simulink model "Simulator_BlockDiagram"  (R2020a)
settings: Solver=FixedStepAuto  StartTime=0.0  StopTime=20  FixedStep=dt  RelTol=1e-3
values from neighbouring files (symbols this model uses):
  Beq = 60    [SimulationParam.m]    (also in SimulationParameters.m; abc_ws.mat; kalmanSS.m; kalmanSSHumInput.m)
  damping_d = 0.001    [SimulationParam.m]    (also in SimulationParameters.m; abc_ws.mat = 0.770835010154; kalmanSSHumInput.m = 0.9)
  dt = 0.001    [SimulationParam.m]    (also in SimulationParameters.m; kalmanSS.m; kalmanSSHumInput.m)
  epos_Ki = 1.190    (= 1.19)    [SimulationParam.m]    (also in SimulationParameters.m; abc_ws.mat; kalmanSSHumInput.m)
  epos_Kp = 11.900    (= 11.9)    [SimulationParam.m]    (also in SimulationParameters.m; abc_ws.mat; kalmanSSHumInput.m)
  Ja = 0.47    [SimulationParam.m]    (also in SimulationParameters.m; abc_ws.mat; kalmanSS.m; kalmanSSHumInput.m)
  Je = W*Le^2    (= 0.88498313856)    [SimulationParam.m]    (also in SimulationParameters.m; abc_ws.mat; kalmanSS.m; kalmanSSHumInput.m)
  Jh = 0.0437    [SimulationParam.m]    (also in SimulationParameters.m; abc_ws.mat; kalmanSS.m; kalmanSSHumInput.m)
  k_bar = 1 - stiffness_d/Ks    (= 0.993269230769)    [SimulationParam.m]    (also in SimulationParameters.m)
  Ka = Ks/20    (= 5.2)    [SimulationParam.m]    (also in SimulationParameters.m; abc_ws.mat = 1387.6; kalmanSS.m = 1387.6; kalmanSSHumInput.m = 800)
  Ks = 104    [SimulationParam.m]    (also in SimulationParameters.m; abc_ws.mat; kalmanSS.m; kalmanSSHumInput.m)
  Le = 0.432    [SimulationParam.m]    (also in SimulationParameters.m; abc_ws.mat; kalmanSS.m; kalmanSSHumInput.m)
  stiffness_d = 0.7    [SimulationParam.m]    (also in SimulationParameters.m; abc_ws.mat = 14.0803237251; kalmanSSHumInput.m = 3.874)
  We = W*g    (= 46.5037717323)    [SimulationParam.m]    (also in SimulationParameters.m; abc_ws.mat; kalmanSS.m; kalmanSSHumInput.m)
libraries: simulink x4, simulink_extras x2, dspstat3 x1
settings Model: Creator=leona  LastModifiedBy=leona
settings DataIOCC: SaveFormat=StructureWithTime  SaveOutput=off  SignalLogging=off  DSMLogging=off  SaveTime=off  ReturnWorkspaceOutputs=off

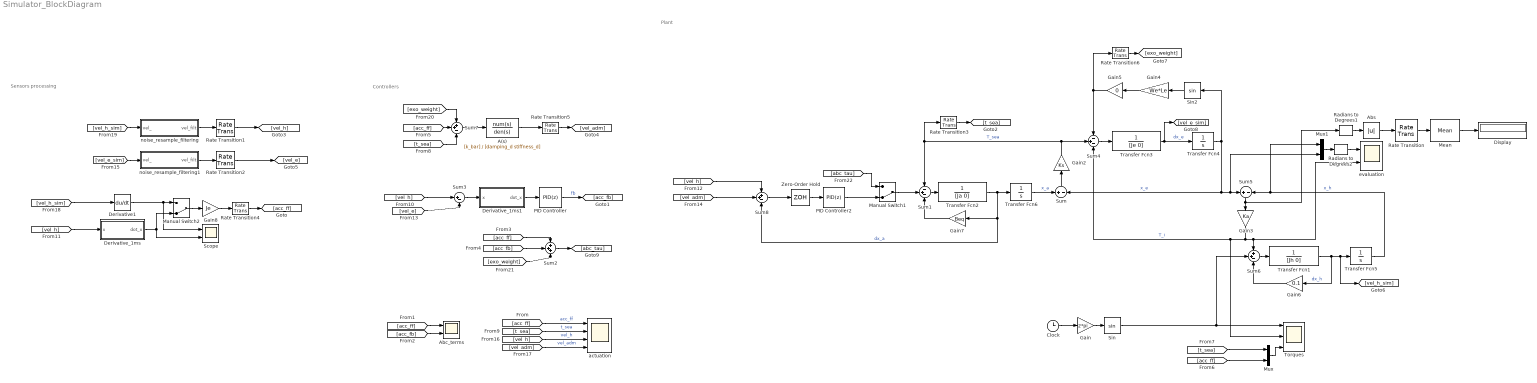
== system Simulator_BlockDiagram ==
  note: Plant
  note: Controllers
  note: Sensors processing
  A(s) : TransferFcn  Numerator=[k_bar]  Denominator=[damping_d stiffness_d]
  Abc_terms : Scope  NumInputPorts=2
  Abs : Abs
  Clock : Clock
  Derivative1 : Derivative
  Derivative_1ms : Subsystem
  Derivative_1ms1 : Subsystem
  Display : Display
  Gain : Gain  Gain=2*pi
  Gain2 : Gain  Gain=Ks
  Gain3 : Gain  Gain=Ka
  Gain4 : Gain  Gain=We*Le
  Gain5 : Gain  Gain=0
  Gain6 : Gain  Gain=0.1
  Gain7 : Gain  Gain=Beq
  Gain8 : Gain  Gain=Je
  Manual Switch1 : ManualSwitch  CurrentSetting=0
  Manual Switch2 : ManualSwitch  CurrentSetting=0
  Mean : dspstat3/Mean  run=on  InputProcessing=Columns as channels (frame based)  reset_popup=None  directionMode=Each column  dimension=1  roiEnable=off  roiType=Rectangles  roiPortion=Entire ROI  roiOutput=Individual statistics for each ROI  roiFlag=off  roundingMode=Floor  overflowMode=off  outputDataTypeStr=Inherit: Same as accumulator  outputMin=[]  outputMax=[]  outputLastDataTypeStr=Inherit: Same as accumulator
  Mux : Mux  Inputs=2
  Mux1 : Mux  Inputs=2
  PID Controller : simulink/Continuous/PID Controller  Controller=PID  Form=Parallel  TimeDomain=Discrete-time  UseExternalTs=off  SampleTime=dt  IntegratorMethod=Forward Euler  FilterMethod=Forward Euler  ControllerParametersSource=internal  P=.1  I=0  D=.01  UseFilter=off  N=100  TunerSelectOption=Transfer Function Based (PID Tuner App)  InitialConditionSource=internal  InitialConditionForIntegrator=0  InitialConditionForFilter=0  DifferentiatorICPrevScaledInput=0  ExternalReset=none  TrackingMode=off  Kt=1  LimitOutput=off  UpperSaturationLimit=inf  LowerSaturationLimit=-inf  LinearizeAsGain=on  AntiWindupMode=none  Kb=1  POutMin=[]  POutMax=[]  IOutMin=[]  IOutMax=[]  DOutMin=[]  DOutMax=[]  NOutMin=[]  NOutMax=[]  SumOutMin=[]  SumOutMax=[]  SaturationOutMin=[]  SaturationOutMax=[]  PParamMin=[]  PParamMax=[]  IParamMin=[]  IParamMax=[]  DParamMin=[]  DParamMax=[]  NParamMin=[]  NParamMax=[]  KbParamMin=[]  KbParamMax=[]  KtParamMin=[]  KtParamMax=[]  KbOutMin=[]  KbOutMax=[]  KtOutMin=[]  KtOutMax=[]  IntegratorOutMin=[]  IntegratorOutMax=[]  FilterOutMin=[]  FilterOutMax=[]  SumI1OutMin=[]  SumI1OutMax=[]  SumI2OutMin=[]  SumI2OutMax=[]  SumI3OutMin=[]  SumI3OutMax=[]  SumI4OutMin=[]  SumI4OutMax=[]  SumDOutMin=[]  SumDOutMax=[]  DifferentiatorOutMin=[]  DifferentiatorOutMax=[]  FilterDiffOutCoefMin=[]  FilterDiffOutCoefMax=[]  ReciprocalOutMin=[]  ReciprocalOutMax=[]  SumDenOutMin=[]  SumDenOutMax=[]  SumNumOutMin=[]  SumNumOutMax=[]  DivideOutMin=[]  DivideOutMax=[]  UdiffTsProdOutMin=[]  UdiffTsProdOutMax=[]  NTsProdOutMin=[]  NTsProdOutMax=[]  UintegralTsProdOutMin=[]  UintegralTsProdOutMax=[]  UngainTsProdOutMin=[]  UngainTsProdOutMax=[]  IntegratorContinuousStateAttributes=''  IntegratorStateMustResolveToSignalObject=off  IntegratorRTWStateStorageClass=Auto  FilterContinuousStateAttributes=''  FilterStateMustResolveToSignalObject=off  FilterRTWStateStorageClass=Auto  ParallelPVariant=InternalParameters  IdealPVariant=Disabled  IVariant=InternalParameters  DVariant=InternalParameters  IntegratorVariant=Discrete  SatVariant=Disabled  AWVariant=Passthrough  PCopyVariant=Disabled  TRVariant=Disabled  FdbkBlocksVariant=Forward  IdealPFdbkVariant=Disabled  SatFdbkVariant=Disabled  DerivativeFilterVariant=Differentiator  NVariant=Passthrough  NCopyVariant=Disabled_SignalSpec  FilterICVariant=InternalICsDifferentiator  IntegratorICVariant=InternalICs  ExternalResetVariant=Disabled  TRSumVariant=Passthrough  SumFdbkVariant=Disabled  SumVariant=Sum_PID  TsampFilterVariant=InternalTs  TsampNgainVariant=Passthrough  TsampIntegralVariant=Passthrough
  PID Controller2 : simulink/Continuous/PID Controller  Controller=PID  Form=Parallel  TimeDomain=Discrete-time  UseExternalTs=off  SampleTime=dt  IntegratorMethod=Forward Euler  FilterMethod=Forward Euler  ControllerParametersSource=internal  P=epos_Kp  I=epos_Ki  D=0  UseFilter=on  N=100  TunerSelectOption=Transfer Function Based (PID Tuner App)  InitialConditionSource=internal  InitialConditionForIntegrator=0  InitialConditionForFilter=0  DifferentiatorICPrevScaledInput=0  ExternalReset=none  TrackingMode=off  Kt=1  LimitOutput=off  UpperSaturationLimit=inf  LowerSaturationLimit=-inf  LinearizeAsGain=on  AntiWindupMode=none  Kb=1  POutMin=[]  POutMax=[]  IOutMin=[]  IOutMax=[]  DOutMin=[]  DOutMax=[]  NOutMin=[]  NOutMax=[]  SumOutMin=[]  SumOutMax=[]  SaturationOutMin=[]  SaturationOutMax=[]  PParamMin=[]  PParamMax=[]  IParamMin=[]  IParamMax=[]  DParamMin=[]  DParamMax=[]  NParamMin=[]  NParamMax=[]  KbParamMin=[]  KbParamMax=[]  KtParamMin=[]  KtParamMax=[]  KbOutMin=[]  KbOutMax=[]  KtOutMin=[]  KtOutMax=[]  IntegratorOutMin=[]  IntegratorOutMax=[]  FilterOutMin=[]  FilterOutMax=[]  SumI1OutMin=[]  SumI1OutMax=[]  SumI2OutMin=[]  SumI2OutMax=[]  SumI3OutMin=[]  SumI3OutMax=[]  SumI4OutMin=[]  SumI4OutMax=[]  SumDOutMin=[]  SumDOutMax=[]  DifferentiatorOutMin=[]  DifferentiatorOutMax=[]  FilterDiffOutCoefMin=[]  FilterDiffOutCoefMax=[]  ReciprocalOutMin=[]  ReciprocalOutMax=[]  SumDenOutMin=[]  SumDenOutMax=[]  SumNumOutMin=[]  SumNumOutMax=[]  DivideOutMin=[]  DivideOutMax=[]  UdiffTsProdOutMin=[]  UdiffTsProdOutMax=[]  NTsProdOutMin=[]  NTsProdOutMax=[]  UintegralTsProdOutMin=[]  UintegralTsProdOutMax=[]  UngainTsProdOutMin=[]  UngainTsProdOutMax=[]  IntegratorContinuousStateAttributes=''  IntegratorStateMustResolveToSignalObject=off  IntegratorRTWStateStorageClass=Auto  FilterContinuousStateAttributes=''  FilterStateMustResolveToSignalObject=off  FilterRTWStateStorageClass=Auto  ParallelPVariant=InternalParameters  IdealPVariant=Disabled  IVariant=InternalParameters  DVariant=InternalParameters  IntegratorVariant=Discrete  SatVariant=Disabled  AWVariant=Passthrough  PCopyVariant=Disabled  TRVariant=Disabled  FdbkBlocksVariant=Forward  IdealPFdbkVariant=Disabled  SatFdbkVariant=Disabled  DerivativeFilterVariant=ForwardEulerFilter  NVariant=InternalParameters  NCopyVariant=Disabled  FilterICVariant=InternalICsFilter  IntegratorICVariant=InternalICs  ExternalResetVariant=Disabled  TRSumVariant=Passthrough  SumFdbkVariant=Disabled  SumVariant=Sum_PID  TsampFilterVariant=InternalTs  TsampNgainVariant=Passthrough  TsampIntegralVariant=Passthrough
  Radians to Degrees1 : simulink_extras/Transformations/Radians to Degrees
  Radians to Degrees2 : simulink_extras/Transformations/Radians to Degrees
  Rate Transition{,1..6} (7 alike) : RateTransition  OutPortSampleTime=dt
  Scope : Scope  NumInputPorts=2
  Sin : Trigonometry
  Sin2 : Trigonometry
  Sum : Sum  Inputs=+-
  Sum1 : Sum  Inputs=-+-
  Sum2 : Sum  Inputs=+++
  Sum3 : Sum  Inputs=|+-
  Sum4 : Sum  Inputs=-+-
  Sum5 : Sum  Inputs=+-
  Sum6 : Sum  Inputs=++-
  Sum7 : Sum  Inputs=++-
  Sum8 : Sum  Inputs=++-
  Torques : Scope  NumInputPorts=3
  Transfer Fcn1 : TransferFcn  Denominator=[Jh 0]
  Transfer Fcn2 : TransferFcn  Denominator=[Ja 0]
  Transfer Fcn3 : TransferFcn  Denominator=[Je 0]
  Transfer Fcn4 : TransferFcn  Denominator=[1 0]
  Transfer Fcn5 : TransferFcn  Denominator=[1 0]
  Transfer Fcn6 : TransferFcn  Denominator=[1 0]
  Zero-Order Hold : ZeroOrderHold  SampleTime=-1
  actuation : Scope  NumInputPorts=4
  evaluation : Scope  NumInputPorts=2
  noise_resample_filtering : Subsystem
  noise_resample_filtering1 : Subsystem
  wires:
  Transfer Fcn6/1 -> Sum/1  "x_a"
  Derivative1/1 -> Scope/1, Manual Switch2/1
  Sum1/1 -> Transfer Fcn2/1
  Sum/1 -> Gain2/1
  Gain2/1 -> Sum4/2, Rate Transition3/1, Sum1/1  "T_sea"
  Sum3/1 -> Derivative_1ms1/1(x)
  Sum4/1 -> Transfer Fcn3/1
  Transfer Fcn4/1 -> Sin2/1, Mux1/2, Sum5/1, Sum/2  "x_e"
  Sin/1 -> Sum6/2, Torques/1
  Sum6/1 -> Transfer Fcn1/1
  Transfer Fcn5/1 -> Mux1/1, Sum5/2  "x_h"
  Sum5/1 -> Radians to Degrees1/1, Gain3/1
  Gain3/1 -> Sum4/3, Torques/2, Sum6/1, evaluation/2  "T_i"
  Transfer Fcn1/1 -> Gain6/1, [vel_h_sim], Transfer Fcn5/1  "dx_h"
  Manual Switch2/1 -> Gain8/1
  Transfer Fcn2/1 -> Sum8/3, Gain7/1, Transfer Fcn6/1  "dx_a"
  Clock/1 -> Gain/1
  Gain/1 -> Sin/1
  Derivative_1ms1/1(dot_x) -> PID Controller/1
  Mux/1 -> Torques/3
  Sum7/1 -> A(s)/1
  Sum8/1 -> Zero-Order Hold/1
  Gain4/1 -> Gain5/1
  Gain5/1 -> Sum4/1, Rate Transition6/1
  Sin2/1 -> Gain4/1
  A(s)/1 -> Rate Transition5/1
  Gain7/1 -> Sum1/3
  Gain6/1 -> Sum6/3
  Radians to Degrees2/1 -> evaluation/1
  Mux1/1 -> Radians to Degrees2/1
  Radians to Degrees1/1 -> Abs/1
  Abs/1 -> Rate Transition/1
  Rate Transition/1 -> Mean/1
  Mean/1 -> Display/1
  [acc_ff] -> Abc_terms/1
  PID Controller/1 -> [acc_fb]  "fb"
  [acc_fb] -> Abc_terms/2
  [acc_ff] -> Sum2/1
  [acc_fb] -> Sum2/2
  [acc_ff] -> Sum7/2
  [acc_ff] -> Mux/2
  [t_sea] -> Sum7/3
  [t_sea] -> Mux/1
  [acc_ff] -> actuation/1  "acc_ff"
  [t_sea] -> actuation/2  "t_sea"
  [vel_h] -> Sum3/1
  [vel_e] -> Sum3/2
  [vel_adm] -> Sum8/2
  [vel_adm] -> actuation/4  "vel_adm"
  [vel_h] -> actuation/3  "vel_h"
  Transfer Fcn3/1 -> [vel_e_sim], Transfer Fcn4/1  "dx_e"
  Gain8/1 -> Rate Transition4/1
  Derivative_1ms/1(dot_x) -> Scope/2, Manual Switch2/2
  [vel_h] -> Sum8/1
  [vel_h] -> Derivative_1ms/1(x)
  noise_resample_filtering/1(vel_filt) -> Rate Transition1/1
  Rate Transition1/1 -> [vel_h]
  noise_resample_filtering1/1(vel_filt) -> Rate Transition2/1
  Rate Transition2/1 -> [vel_e]
  [vel_h_sim] -> Derivative1/1
  [vel_e_sim] -> noise_resample_filtering1/1(vel_)
  [vel_h_sim] -> noise_resample_filtering/1(vel_)
  Rate Transition3/1 -> [t_sea]
  Rate Transition4/1 -> [acc_ff]
  Rate Transition5/1 -> [vel_adm]
  [exo_weight] -> Sum7/1
  Rate Transition6/1 -> [exo_weight]
  Zero-Order Hold/1 -> PID Controller2/1
  Manual Switch1/1 -> Sum1/2
  PID Controller2/1 -> Manual Switch1/2
  [exo_weight] -> Sum2/3
  Sum2/1 -> [abc_tau]
  [abc_tau] -> Manual Switch1/1

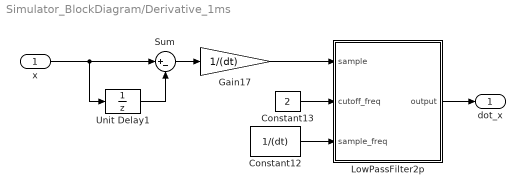
== system Simulator_BlockDiagram/Derivative_1ms ==
  x : Inport
  Constant12 : Constant  Value=1/(dt)
  Constant13 : Constant  Value=2
  Gain17 : Gain  Gain=1/(dt)
  LowPassFilter2p : Subsystem
  Sum : Sum  Inputs=|+-
  Unit Delay1 : UnitDelay  SampleTime=-1  HasFrameUpgradeWarning=on
  dot_x : Outport
  wires:
  Unit Delay1/1 -> Sum/2
  Sum/1 -> Gain17/1
  Gain17/1 -> LowPassFilter2p/1(sample)
  LowPassFilter2p/1(output) -> dot_x/1
  Constant12/1 -> LowPassFilter2p/3(sample_freq)
  x/1 -> Unit Delay1/1, Sum/1
  Constant13/1 -> LowPassFilter2p/2(cutoff_freq)

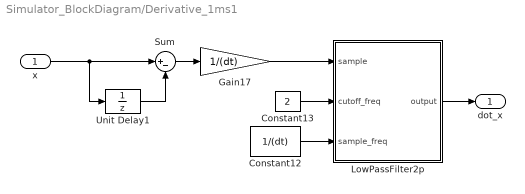
== system Simulator_BlockDiagram/Derivative_1ms1 ==
  x : Inport
  Constant12 : Constant  Value=1/(dt)
  Constant13 : Constant  Value=2
  Gain17 : Gain  Gain=1/(dt)
  LowPassFilter2p : Subsystem
  Sum : Sum  Inputs=|+-
  Unit Delay1 : UnitDelay  SampleTime=-1  HasFrameUpgradeWarning=on
  dot_x : Outport
  wires:
  Constant13/1 -> LowPassFilter2p/2(cutoff_freq)
  x/1 -> Sum/1, Unit Delay1/1
  Constant12/1 -> LowPassFilter2p/3(sample_freq)
  LowPassFilter2p/1(output) -> dot_x/1
  Gain17/1 -> LowPassFilter2p/1(sample)
  Sum/1 -> Gain17/1
  Unit Delay1/1 -> Sum/2

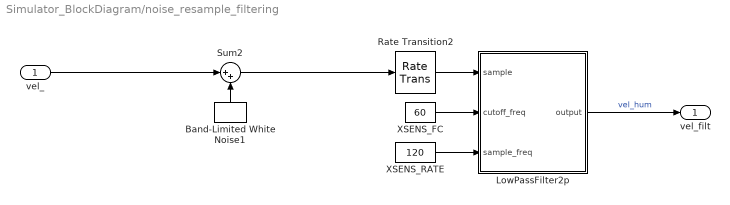
== system Simulator_BlockDiagram/noise_resample_filtering ==
  vel_ : Inport
  Band-Limited White Noise1 : simulink/Sources/Band-Limited White Noise  Cov=[dt*dt*0.3]  Ts=dt  seed=[48236]  VectorParams1D=off
  LowPassFilter2p : Subsystem
  Rate Transition2 : RateTransition  OutPortSampleTime=0.008
  Sum2 : Sum  Inputs=|++
  XSENS_FC : Constant  Value=60
  XSENS_RATE : Constant  Value=120
  vel_filt : Outport
  wires:
  vel_/1 -> Sum2/1
  XSENS_FC/1 -> LowPassFilter2p/2(cutoff_freq)
  LowPassFilter2p/1(output) -> vel_filt/1  "vel_hum"
  Sum2/1 -> Rate Transition2/1
  Band-Limited White Noise1/1 -> Sum2/2
  Rate Transition2/1 -> LowPassFilter2p/1(sample)
  XSENS_RATE/1 -> LowPassFilter2p/3(sample_freq)

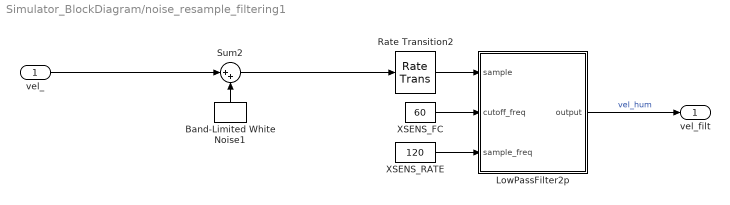
== system Simulator_BlockDiagram/noise_resample_filtering1 ==
  vel_ : Inport
  Band-Limited White Noise1 : simulink/Sources/Band-Limited White Noise  Cov=[dt*dt*0.3]  Ts=dt  seed=[48236]  VectorParams1D=off
  LowPassFilter2p : Subsystem
  Rate Transition2 : RateTransition  OutPortSampleTime=0.008
  Sum2 : Sum  Inputs=|++
  XSENS_FC : Constant  Value=60
  XSENS_RATE : Constant  Value=120
  vel_filt : Outport
  wires:
  XSENS_RATE/1 -> LowPassFilter2p/3(sample_freq)
  Rate Transition2/1 -> LowPassFilter2p/1(sample)
  Band-Limited White Noise1/1 -> Sum2/2
  Sum2/1 -> Rate Transition2/1
  LowPassFilter2p/1(output) -> vel_filt/1  "vel_hum"
  XSENS_FC/1 -> LowPassFilter2p/2(cutoff_freq)
  vel_/1 -> Sum2/1

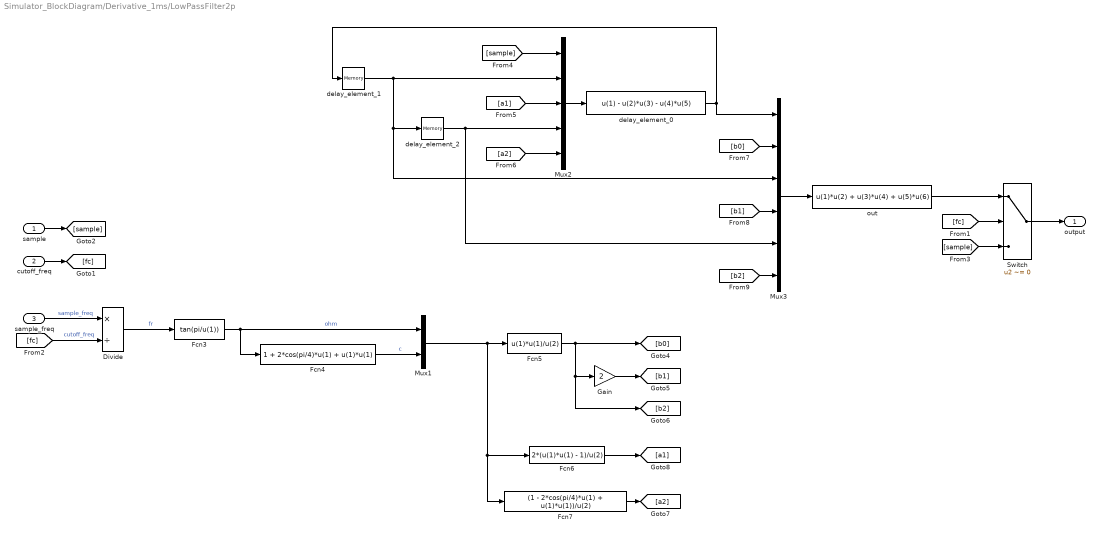
== system Simulator_BlockDiagram/Derivative_1ms/LowPassFilter2p ==
  sample : Inport
  cutoff_freq : Inport  Port=2
  sample_freq : Inport  Port=3
  Divide : Product  Inputs=*/
  Fcn3 : Fcn  Expr=tan(pi/u(1))
  Fcn4 : Fcn  Expr=1 + 2*cos(pi/4)*u(1) + u(1)*u(1)
  Fcn5 : Fcn  Expr=u(1)*u(1)/u(2)
  Fcn6 : Fcn  Expr=2*(u(1)*u(1) - 1)/u(2)
  Fcn7 : Fcn  Expr=(1 - 2*cos(pi/4)*u(1) + u(1)*u(1))/u(2)
  Gain : Gain  Gain=2
  Mux1 : Mux  Inputs=2
  Mux2 : Mux  Inputs=5
  Mux3 : Mux  Inputs=6
  Switch : Switch  Criteria=u2 ~= 0
  delay_element_0 : Fcn  Expr=u(1) - u(2)*u(3) - u(4)*u(5)
  delay_element_1 : Memory  InheritSampleTime=on
  delay_element_2 : Memory  InheritSampleTime=on
  out : Fcn  Expr=u(1)*u(2) + u(3)*u(4) + u(5)*u(6)
  output : Outport
  wires:
  Switch/1 -> output/1
  cutoff_freq/1 -> [fc]
  [fc] -> Switch/2
  sample_freq/1 -> Divide/1  "sample_freq"
  [fc] -> Divide/2  "cutoff_freq"
  Divide/1 -> Fcn3/1  "fr"
  Mux1/1 -> Fcn7/1, Fcn6/1, Fcn5/1
  Fcn3/1 -> Mux1/1, Fcn4/1  "ohm"
  Fcn4/1 -> Mux1/2  "c"
  Fcn5/1 -> [b0], [b2], Gain/1
  Gain/1 -> [b1]
  Fcn6/1 -> [a1]
  Fcn7/1 -> [a2]
  sample/1 -> [sample]
  [sample] -> Switch/3
  delay_element_1/1 -> delay_element_2/1, Mux3/3, Mux2/2
  [sample] -> Mux2/1
  Mux2/1 -> delay_element_0/1
  [a1] -> Mux2/3
  delay_element_2/1 -> Mux2/4, Mux3/5
  [a2] -> Mux2/5
  out/1 -> Switch/1
  delay_element_0/1 -> delay_element_1/1, Mux3/1
  [b0] -> Mux3/2
  [b1] -> Mux3/4
  [b2] -> Mux3/6
  Mux3/1 -> out/1

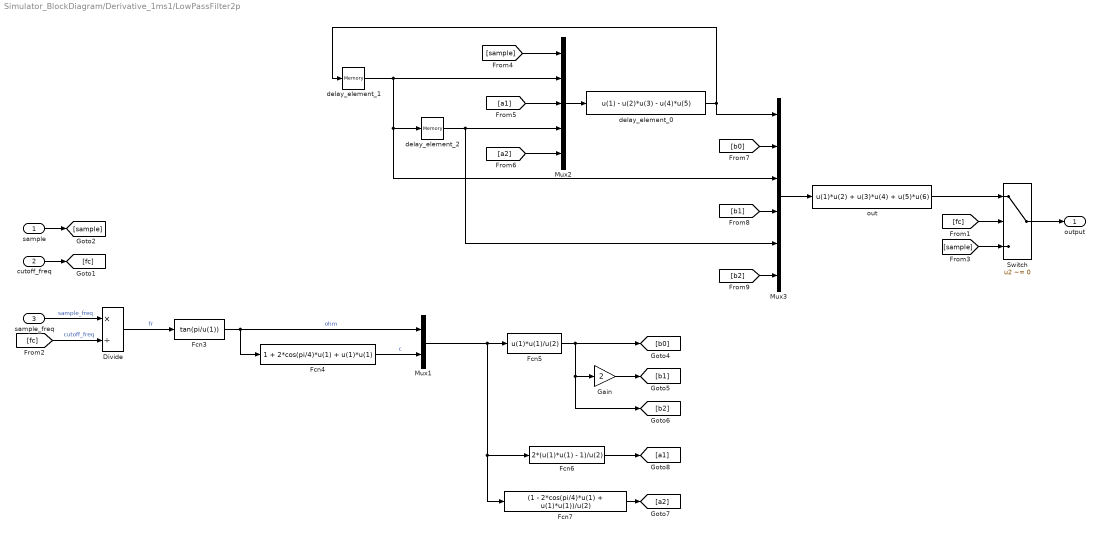
== system Simulator_BlockDiagram/Derivative_1ms1/LowPassFilter2p ==
  sample : Inport
  cutoff_freq : Inport  Port=2
  sample_freq : Inport  Port=3
  Divide : Product  Inputs=*/
  Fcn3 : Fcn  Expr=tan(pi/u(1))
  Fcn4 : Fcn  Expr=1 + 2*cos(pi/4)*u(1) + u(1)*u(1)
  Fcn5 : Fcn  Expr=u(1)*u(1)/u(2)
  Fcn6 : Fcn  Expr=2*(u(1)*u(1) - 1)/u(2)
  Fcn7 : Fcn  Expr=(1 - 2*cos(pi/4)*u(1) + u(1)*u(1))/u(2)
  Gain : Gain  Gain=2
  Mux1 : Mux  Inputs=2
  Mux2 : Mux  Inputs=5
  Mux3 : Mux  Inputs=6
  Switch : Switch  Criteria=u2 ~= 0
  delay_element_0 : Fcn  Expr=u(1) - u(2)*u(3) - u(4)*u(5)
  delay_element_1 : Memory  InheritSampleTime=on
  delay_element_2 : Memory  InheritSampleTime=on
  out : Fcn  Expr=u(1)*u(2) + u(3)*u(4) + u(5)*u(6)
  output : Outport
  wires:
  Mux3/1 -> out/1
  [b2] -> Mux3/6
  [b1] -> Mux3/4
  [b0] -> Mux3/2
  delay_element_0/1 -> Mux3/1, delay_element_1/1
  out/1 -> Switch/1
  [a2] -> Mux2/5
  delay_element_2/1 -> Mux3/5, Mux2/4
  [a1] -> Mux2/3
  Mux2/1 -> delay_element_0/1
  [sample] -> Mux2/1
  delay_element_1/1 -> Mux2/2, Mux3/3, delay_element_2/1
  [sample] -> Switch/3
  sample/1 -> [sample]
  Fcn7/1 -> [a2]
  Fcn6/1 -> [a1]
  Gain/1 -> [b1]
  Fcn5/1 -> Gain/1, [b2], [b0]
  Fcn4/1 -> Mux1/2  "c"
  Fcn3/1 -> Fcn4/1, Mux1/1  "ohm"
  Mux1/1 -> Fcn5/1, Fcn6/1, Fcn7/1
  Divide/1 -> Fcn3/1  "fr"
  [fc] -> Divide/2  "cutoff_freq"
  sample_freq/1 -> Divide/1  "sample_freq"
  [fc] -> Switch/2
  cutoff_freq/1 -> [fc]
  Switch/1 -> output/1

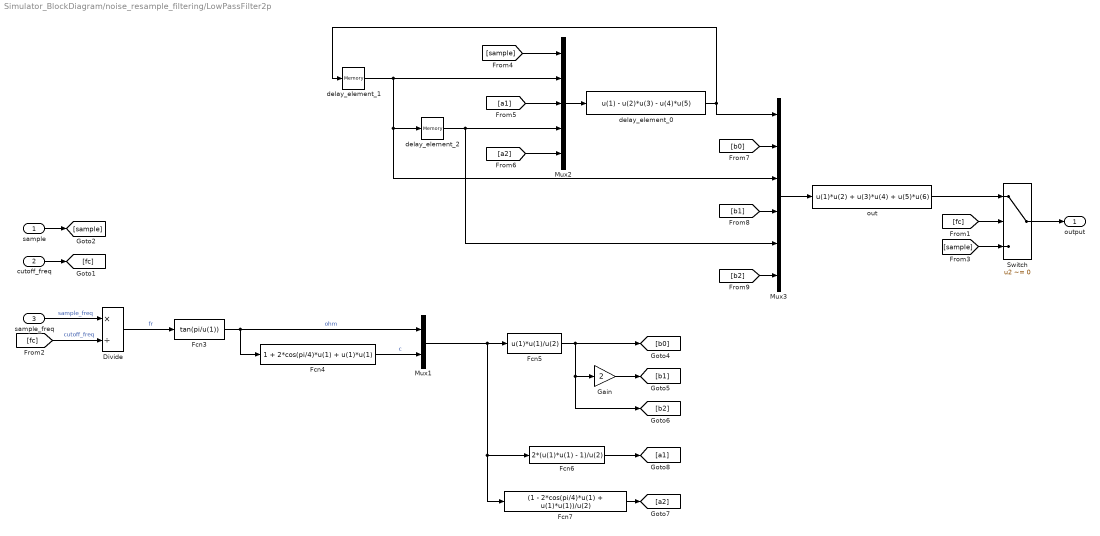
== system Simulator_BlockDiagram/noise_resample_filtering/LowPassFilter2p ==
  sample : Inport
  cutoff_freq : Inport  Port=2
  sample_freq : Inport  Port=3
  Divide : Product  Inputs=*/
  Fcn3 : Fcn  Expr=tan(pi/u(1))
  Fcn4 : Fcn  Expr=1 + 2*cos(pi/4)*u(1) + u(1)*u(1)
  Fcn5 : Fcn  Expr=u(1)*u(1)/u(2)
  Fcn6 : Fcn  Expr=2*(u(1)*u(1) - 1)/u(2)
  Fcn7 : Fcn  Expr=(1 - 2*cos(pi/4)*u(1) + u(1)*u(1))/u(2)
  Gain : Gain  Gain=2
  Mux1 : Mux  Inputs=2
  Mux2 : Mux  Inputs=5
  Mux3 : Mux  Inputs=6
  Switch : Switch  Criteria=u2 ~= 0
  delay_element_0 : Fcn  Expr=u(1) - u(2)*u(3) - u(4)*u(5)
  delay_element_1 : Memory  InheritSampleTime=on
  delay_element_2 : Memory  InheritSampleTime=on
  out : Fcn  Expr=u(1)*u(2) + u(3)*u(4) + u(5)*u(6)
  output : Outport
  wires:
  Switch/1 -> output/1
  cutoff_freq/1 -> [fc]
  [fc] -> Switch/2
  sample_freq/1 -> Divide/1  "sample_freq"
  [fc] -> Divide/2  "cutoff_freq"
  Divide/1 -> Fcn3/1  "fr"
  Mux1/1 -> Fcn7/1, Fcn6/1, Fcn5/1
  Fcn3/1 -> Mux1/1, Fcn4/1  "ohm"
  Fcn4/1 -> Mux1/2  "c"
  Fcn5/1 -> [b0], [b2], Gain/1
  Gain/1 -> [b1]
  Fcn6/1 -> [a1]
  Fcn7/1 -> [a2]
  sample/1 -> [sample]
  [sample] -> Switch/3
  delay_element_1/1 -> delay_element_2/1, Mux3/3, Mux2/2
  [sample] -> Mux2/1
  Mux2/1 -> delay_element_0/1
  [a1] -> Mux2/3
  delay_element_2/1 -> Mux2/4, Mux3/5
  [a2] -> Mux2/5
  out/1 -> Switch/1
  delay_element_0/1 -> delay_element_1/1, Mux3/1
  [b0] -> Mux3/2
  [b1] -> Mux3/4
  [b2] -> Mux3/6
  Mux3/1 -> out/1

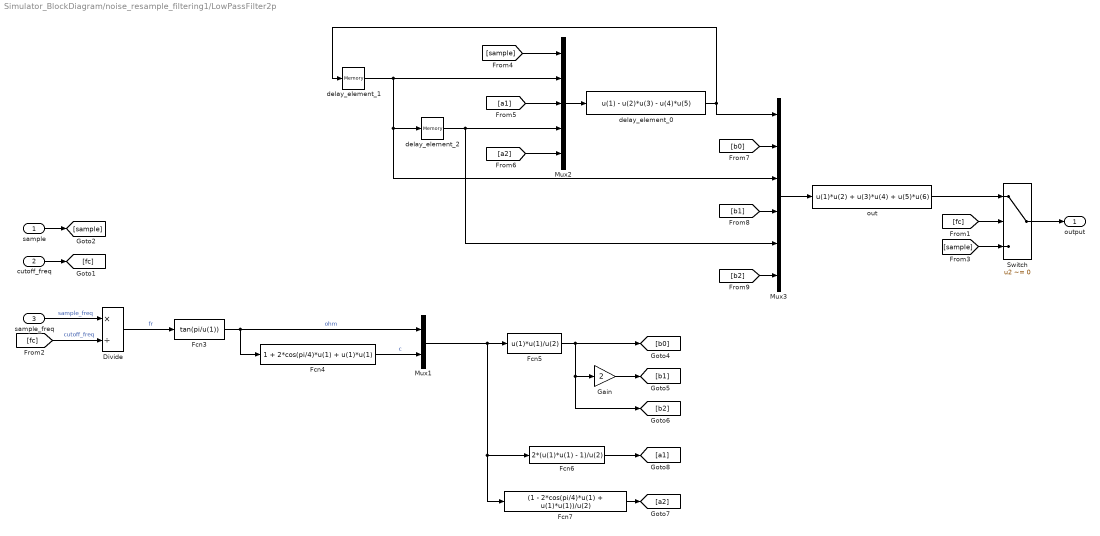
== system Simulator_BlockDiagram/noise_resample_filtering1/LowPassFilter2p ==
  sample : Inport
  cutoff_freq : Inport  Port=2
  sample_freq : Inport  Port=3
  Divide : Product  Inputs=*/
  Fcn3 : Fcn  Expr=tan(pi/u(1))
  Fcn4 : Fcn  Expr=1 + 2*cos(pi/4)*u(1) + u(1)*u(1)
  Fcn5 : Fcn  Expr=u(1)*u(1)/u(2)
  Fcn6 : Fcn  Expr=2*(u(1)*u(1) - 1)/u(2)
  Fcn7 : Fcn  Expr=(1 - 2*cos(pi/4)*u(1) + u(1)*u(1))/u(2)
  Gain : Gain  Gain=2
  Mux1 : Mux  Inputs=2
  Mux2 : Mux  Inputs=5
  Mux3 : Mux  Inputs=6
  Switch : Switch  Criteria=u2 ~= 0
  delay_element_0 : Fcn  Expr=u(1) - u(2)*u(3) - u(4)*u(5)
  delay_element_1 : Memory  InheritSampleTime=on
  delay_element_2 : Memory  InheritSampleTime=on
  out : Fcn  Expr=u(1)*u(2) + u(3)*u(4) + u(5)*u(6)
  output : Outport
  wires:
  Mux3/1 -> out/1
  [b2] -> Mux3/6
  [b1] -> Mux3/4
  [b0] -> Mux3/2
  delay_element_0/1 -> Mux3/1, delay_element_1/1
  out/1 -> Switch/1
  [a2] -> Mux2/5
  delay_element_2/1 -> Mux3/5, Mux2/4
  [a1] -> Mux2/3
  Mux2/1 -> delay_element_0/1
  [sample] -> Mux2/1
  delay_element_1/1 -> Mux2/2, Mux3/3, delay_element_2/1
  [sample] -> Switch/3
  sample/1 -> [sample]
  Fcn7/1 -> [a2]
  Fcn6/1 -> [a1]
  Gain/1 -> [b1]
  Fcn5/1 -> Gain/1, [b2], [b0]
  Fcn4/1 -> Mux1/2  "c"
  Fcn3/1 -> Fcn4/1, Mux1/1  "ohm"
  Mux1/1 -> Fcn5/1, Fcn6/1, Fcn7/1
  Divide/1 -> Fcn3/1  "fr"
  [fc] -> Divide/2  "cutoff_freq"
  sample_freq/1 -> Divide/1  "sample_freq"
  [fc] -> Switch/2
  cutoff_freq/1 -> [fc]
  Switch/1 -> output/1
